simulink model "podd2012B"  (R2012b)
settings: Solver=ode45  StartTime=0.0  StopTime=600  RelTol=1e-3
undefined symbols (not defined in the file): A1, A2, mi1, mi2, mu1
settings Model: Creator=Sandra Knezevic  LastModifiedBy=Aldin
settings OptimizationCC: ExpressionDepthLimit=128
settings DebuggingCC: UnderspecifiedInitializationDetection=Simplified  MergeDetectMultiDrivingBlocksExec=error  SolverPrmCheckMsg=none  FrameProcessingCompatibilityMsg=error  StateNameClashWarn=none
settings CodeAppCC: CustomSymbolStrType=$N$R$M_T
settings GRTTargetCC: CodeReplacementLibrary=C89/C90 (ANSI)

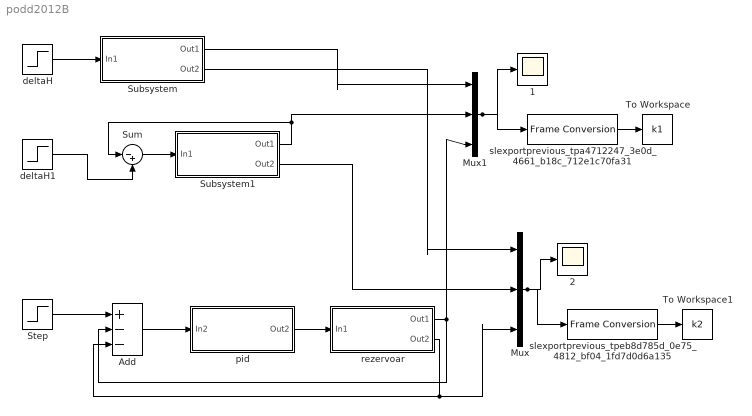
== system podd2012B ==
  1 : Scope
      settings: TimeRange=auto  ShowLegends=on  LimitDataPoints=on  MaxDataPoints=5000  SaveToWorkspace=off  YMin=-10  YMax=10  SampleTime=-1  DataFormat=Array
  2 : Scope
      settings: TimeRange=auto  LimitDataPoints=on  MaxDataPoints=5000  SaveToWorkspace=off  SaveName=ScopeData  YMin=-10  YMax=10  SampleTime=-1  DataFormat=Array
  Add : Sum  Inputs=+--
  Mux : Mux  Inputs=3
  Mux1 : Mux  Inputs=3
  Step : Step  Time=0  Before=1  After=10  SampleTime=0
  Subsystem : Subsystem
  Subsystem1 : Subsystem
  Sum : Sum  Inputs=|-+
  To Workspace : ToWorkspace  VariableName=k1  SampleTime=-1
  To Workspace1 : ToWorkspace  VariableName=k2  SampleTime=-1
  deltaH : Step  After=15  SampleTime=0
  deltaH1 : Step  After=15  SampleTime=0
  pid : Subsystem
  rezervoar : Subsystem
  slexportprevious_tpa4712247_3e0d_4661_b18c_712e1c70fa31 : FrameConversion  OutFrame=Sample-based
  slexportprevious_tpeb8d785d_0e75_4812_bf04_1fd7d0d6a135 : FrameConversion  OutFrame=Sample-based
  wires:
  deltaH/1 -> Subsystem/1(In1)
  deltaH1/1 -> Sum/2
  Sum/1 -> Subsystem1/1(In1)
  Subsystem1/1(Out1) -> Mux1/2, Sum/1
  pid/1(Out2) -> rezervoar/1(In1)
  Add/1 -> pid/1(In2)
  Step/1 -> Add/1
  rezervoar/1(Out1) -> Mux1/3, Add/2
  rezervoar/2(Out2) -> Add/3, Mux/3
  Mux1/1 -> 1/1, slexportprevious_tpa4712247_3e0d_4661_b18c_712e1c70fa31/1
  Subsystem/1(Out1) -> Mux1/1
  Subsystem/2(Out2) -> Mux/1
  Subsystem1/2(Out2) -> Mux/2
  Mux/1 -> 2/1, slexportprevious_tpeb8d785d_0e75_4812_bf04_1fd7d0d6a135/1
  slexportprevious_tpa4712247_3e0d_4661_b18c_712e1c70fa31/1 -> To Workspace/1
  slexportprevious_tpeb8d785d_0e75_4812_bf04_1fd7d0d6a135/1 -> To Workspace1/1

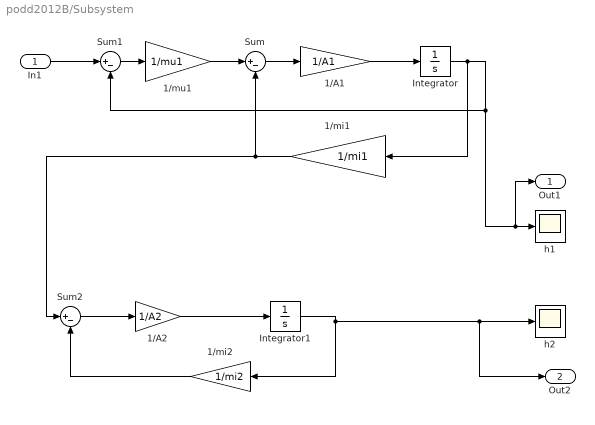
== system podd2012B/Subsystem ==
  In1 : Inport
  1/A1 : Gain  Gain=1/A1
  1/A2 : Gain  Gain=1/A2
  1/mi1 : Gain  Gain=1/mi1
  1/mi2 : Gain  Gain=1/mi2
  1/mu1 : Gain  Gain=1/mu1
  Integrator : Integrator  InitialCondition=1
  Integrator1 : Integrator  InitialCondition=1
  Sum : Sum  Inputs=|+-
  Sum1 : Sum  Inputs=|+-
  Sum2 : Sum  Inputs=|+-
  h1 : Scope
      settings: TimeRange=600  LimitDataPoints=on  MaxDataPoints=5000  SaveToWorkspace=off  SaveName=ScopeData2  YMin=-10  YMax=10  SampleTime=-1  DataFormat=Array
  h2 : Scope
      settings: TimeRange=600  LimitDataPoints=on  MaxDataPoints=5000  SaveToWorkspace=off  SaveName=ScopeData3  YMin=-10  YMax=10  SampleTime=-1  DataFormat=Array
  Out1 : Outport
  Out2 : Outport  Port=2
  wires:
  Integrator1/1 -> Out2/1, h2/1, 1/mi2/1
  Sum/1 -> 1/A1/1
  1/mi2/1 -> Sum2/2
  Sum1/1 -> 1/mu1/1
  1/A2/1 -> Integrator1/1
  1/mu1/1 -> Sum/1
  1/mi1/1 -> Sum/2, Sum2/1
  In1/1 -> Sum1/1
  Integrator/1 -> 1/mi1/1, Out1/1, h1/1, Sum1/2
  1/A1/1 -> Integrator/1
  Sum2/1 -> 1/A2/1

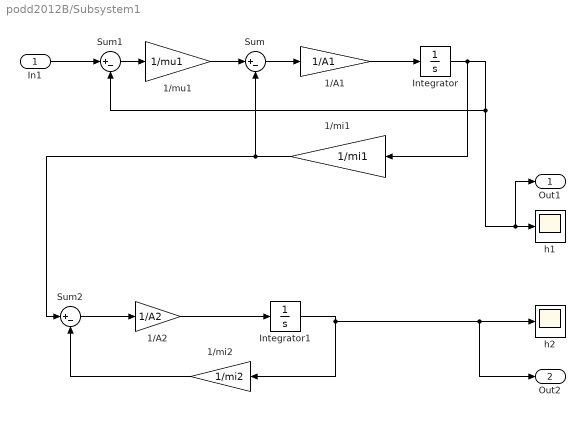
== system podd2012B/Subsystem1 ==
  In1 : Inport
  1/A1 : Gain  Gain=1/A1
  1/A2 : Gain  Gain=1/A2
  1/mi1 : Gain  Gain=1/mi1
  1/mi2 : Gain  Gain=1/mi2
  1/mu1 : Gain  Gain=1/mu1
  Integrator : Integrator  InitialCondition=1
  Integrator1 : Integrator  InitialCondition=1
  Sum : Sum  Inputs=|+-
  Sum1 : Sum  Inputs=|+-
  Sum2 : Sum  Inputs=|+-
  h1 : Scope
      settings: TimeRange=600  LimitDataPoints=on  MaxDataPoints=5000  SaveToWorkspace=off  SaveName=ScopeData4  YMin=-10  YMax=10  SampleTime=-1  DataFormat=Array
  h2 : Scope
      settings: TimeRange=600  LimitDataPoints=on  MaxDataPoints=5000  SaveToWorkspace=off  SaveName=ScopeData5  YMin=-10  YMax=10  SampleTime=-1  DataFormat=Array
  Out1 : Outport
  Out2 : Outport  Port=2
  wires:
  Sum2/1 -> 1/A2/1
  1/A1/1 -> Integrator/1
  1/mi1/1 -> Sum/2, Sum2/1
  1/mu1/1 -> Sum/1
  Sum1/1 -> 1/mu1/1
  1/A2/1 -> Integrator1/1
  1/mi2/1 -> Sum2/2
  Integrator/1 -> 1/mi1/1, Out1/1, h1/1, Sum1/2
  In1/1 -> Sum1/1
  Integrator1/1 -> Out2/1, h2/1, 1/mi2/1
  Sum/1 -> 1/A1/1

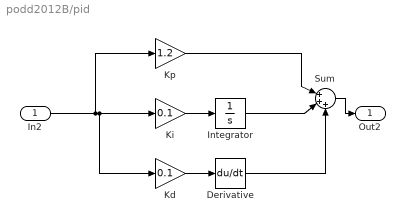
== system podd2012B/pid ==
  In2 : Inport
  Derivative : Derivative
  Integrator : Integrator
  Kd : Gain  Gain=0.1
  Ki : Gain  Gain=0.1
  Kp : Gain  Gain=1.2
  Sum : Sum  Inputs=|+++
  Out2 : Outport
  wires:
  Kp/1 -> Sum/1
  Integrator/1 -> Sum/2
  Derivative/1 -> Sum/3
  Sum/1 -> Out2/1
  In2/1 -> Kp/1, Kd/1, Ki/1
  Ki/1 -> Integrator/1
  Kd/1 -> Derivative/1

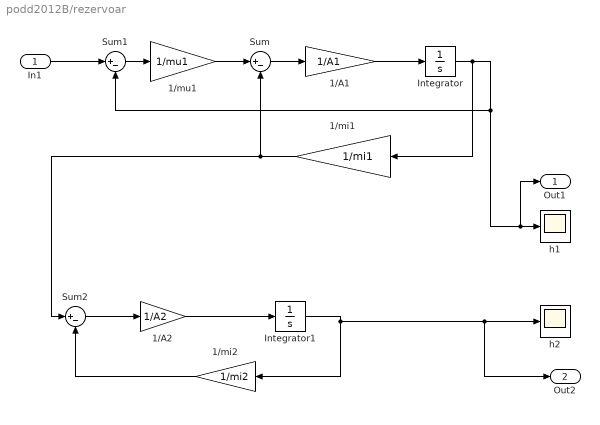
== system podd2012B/rezervoar ==
  In1 : Inport
  1/A1 : Gain  Gain=1/A1
  1/A2 : Gain  Gain=1/A2
  1/mi1 : Gain  Gain=1/mi1
  1/mi2 : Gain  Gain=1/mi2
  1/mu1 : Gain  Gain=1/mu1
  Integrator : Integrator  InitialCondition=1
  Integrator1 : Integrator  InitialCondition=1
  Sum : Sum  Inputs=|+-
  Sum1 : Sum  Inputs=|+-
  Sum2 : Sum  Inputs=|+-
  h1 : Scope
      settings: TimeRange=600  LimitDataPoints=on  MaxDataPoints=5000  SaveToWorkspace=off  SaveName=ScopeData6  YMin=-10  YMax=10  SampleTime=-1  DataFormat=Array
  h2 : Scope
      settings: TimeRange=600  LimitDataPoints=on  MaxDataPoints=5000  SaveToWorkspace=off  SaveName=ScopeData7  YMin=-10  YMax=10  SampleTime=-1  DataFormat=Array
  Out1 : Outport
  Out2 : Outport  Port=2
  wires:
  Sum2/1 -> 1/A2/1
  1/A1/1 -> Integrator/1
  1/mi1/1 -> Sum/2, Sum2/1
  1/mu1/1 -> Sum/1
  Sum1/1 -> 1/mu1/1
  1/A2/1 -> Integrator1/1
  1/mi2/1 -> Sum2/2
  Integrator/1 -> 1/mi1/1, Out1/1, h1/1, Sum1/2
  In1/1 -> Sum1/1
  Integrator1/1 -> Out2/1, h2/1, 1/mi2/1
  Sum/1 -> 1/A1/1
